simulink model "Lecture1Pendulum"  (R2020b)
settings: Solver=VariableStepAuto  StartTime=0.0  StopTime=10  RelTol=1e-3
values from neighbouring files (symbols this model uses):
  g = 9.82    [Lecture1Pendulum.m]
  J = 0.1    [Lecture10_11Exercise.m]    (also in Lecture1Pendulum.m = 0.9; Lecture6Exercise.m)
  L = 1    [Lecture1Pendulum.m]    (also in Lecture5Exercises.m = acker(A_bb', A_ab', [zper zper])')
  m = m_gram/1000    (= 0.9)    [Lecture1Pendulum.m]
  Tf = 0.5    [Lecture1Pendulum.m]
settings Model: Creator=sebastian  LastModifiedBy=sebastian

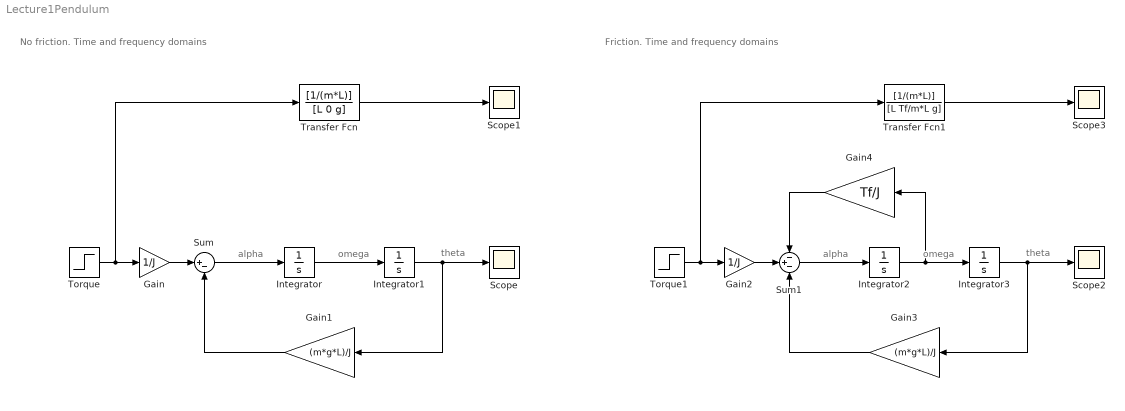
== system Lecture1Pendulum ==
  note: No friction. Time and frequency domains
  note: theta
  note: omega
  note: alpha
  note: alpha
  note: Friction. Time and frequency domains
  note: omega
  note: theta
  Gain : Gain  Gain=1/J
  Gain1 : Gain  Gain=(m*g*L)/J
  Gain2 : Gain  Gain=1/J
  Gain3 : Gain  Gain=(m*g*L)/J
  Gain4 : Gain  Gain=Tf/J
  Integrator{,1..3} (4 alike) : Integrator
  Scope{,1..3} (4 alike) : Scope
  Sum : Sum  Inputs=|+-
  Sum1 : Sum  Inputs=-+-
  Torque : Step  SampleTime=0
  Torque1 : Step  SampleTime=0
  Transfer Fcn : TransferFcn  Numerator=[1/(m*L)]  Denominator=[L 0 g]
  Transfer Fcn1 : TransferFcn  Numerator=[1/(m*L)]  Denominator=[L Tf/m*L g]
  wires:
  Torque/1 -> Transfer Fcn/1, Gain/1
  Gain/1 -> Sum/1
  Sum/1 -> Integrator/1
  Integrator/1 -> Integrator1/1
  Integrator1/1 -> Gain1/1, Scope/1
  Gain1/1 -> Sum/2
  Transfer Fcn/1 -> Scope1/1
  Integrator3/1 -> Gain3/1, Scope2/1
  Integrator2/1 -> Gain4/1, Integrator3/1
  Torque1/1 -> Transfer Fcn1/1, Gain2/1
  Transfer Fcn1/1 -> Scope3/1
  Sum1/1 -> Integrator2/1
  Gain4/1 -> Sum1/1
  Gain2/1 -> Sum1/2
  Gain3/1 -> Sum1/3
